simulink model "FF_statefbk"  (R2020b)
settings: Solver=ode45  StartTime=0.0  StopTime=10  RelTol=1e-3  EnableMultiTasking=on
values from neighbouring files (symbols this model uses):
  A = [0 1 ... (first row only)    [TestDIST_EFFECT_DCmotor_zp(1).m]    (also in TestDIST_EFFECT_DCmotor_zp.m; lqr_DOB_2_5.mat = [0  1; 0  0]; lqr_DOB_5.mat = [0  1; 0  0]; lqr_DOB_8.mat = [0  1; 0  0])
  B = [0; Kt/Rm/Jt]    [TestDIST_EFFECT_DCmotor_zp(1).m]    (also in TestDIST_EFFECT_DCmotor_zp.m; lqr_DOB_2_5.mat = [0 239.250934036]; lqr_DOB_5.mat = [0 239.250934036]; lqr_DOB_8.mat = [0 239.250934036])
  Jt = Jm+J1+J2    (= 2.089856e-05)    [TestDIST_EFFECT_DCmotor_zp(1).m]    (also in TestDIST_EFFECT_DCmotor_zp.m; lqr_DOB_2_5.mat; lqr_DOB_5.mat; lqr_DOB_8.mat)
  KK = dlqr(Fs,Gs,Q,R)    [TestDIST_EFFECT_DCmotor_zp(1).m]    (also in TestDIST_EFFECT_DCmotor_zp.m; lqr_DOB_2_5.mat = [27.9647466006 0.483496818901]; lqr_DOB_5.mat = [27.9647466006 0.483496818901]; lqr_DOB_8.mat = [27.9647466006 0.483496818901])
  Kt = 0.042    [TestDIST_EFFECT_DCmotor_zp(1).m]    (also in TestDIST_EFFECT_DCmotor_zp.m; lqr_DOB_2_5.mat; lqr_DOB_5.mat; lqr_DOB_8.mat)
  Rm = 8.4    [TestDIST_EFFECT_DCmotor_zp(1).m]    (also in TestDIST_EFFECT_DCmotor_zp.m; lqr_DOB_2_5.mat; lqr_DOB_5.mat; lqr_DOB_8.mat)
settings Model: Creator=oboe  LastModifiedBy=marco
settings DataIOCC: LimitDataPoints=on  SaveFormat=Array  ReturnWorkspaceOutputs=off
settings OptimizationCC: LifeSpan=inf
settings DebuggingCC: SolverPrmCheckMsg=warning  SFUnexpectedBacktrackingDiag=warning  SFNoUnconditionalDefaultTransitionDiag=warning  SFExecutionAtInitializationDiag=none  ArithmeticOperatorsInVariantConditions=warning
settings HardwareCC: ProdBitPerPointer=32  ProdBitPerSizeT=32  ProdBitPerPtrDiffT=32  ProdLargestAtomicFloat=None  ProdIntDivRoundTo=Undefined  ProdEndianess=Unspecified  ProdWordSize=32  ProdHWDeviceType=32-bit Generic
settings ModelReferenceCC: PropagateSignalLabelsOutOfModel=off
settings SFSimCC: SimUseLocalCustomCode=off  CustomCodeUndefinedFunction=UseInterfaceOnly
settings RTWCC: RTWUseLocalCustomCode=off
settings CodeAppCC: StateflowObjectComments=on
settings GRTTargetCC: TargetLangStandard=C89/C90 (ANSI)
settings ConfigComp: CovMetricSettings=dw  CovSaveCumulativeToWorkspaceVar=on  CovSaveSingleToWorkspaceVar=on  CovExternalEMLEnable=off  CovSFcnEnable=off

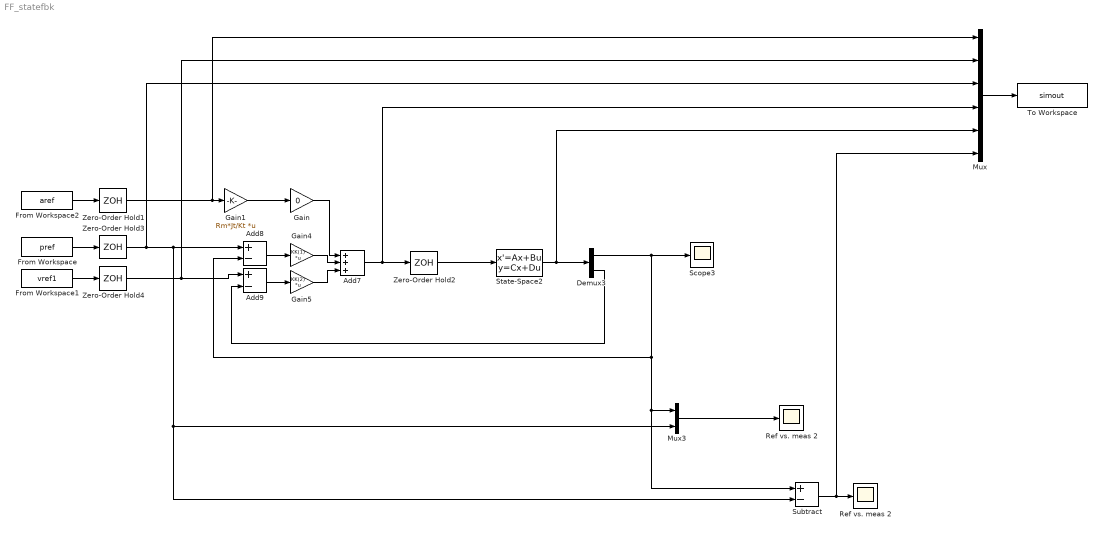
== system FF_statefbk ==
  Add7 : Sum  Inputs=+++
  Add8 : Sum  Inputs=+-
  Add9 : Sum  Inputs=+-
  Demux3 : Demux  Outputs=2
  From Workspace : FromWorkspace  VariableName=pref
  From Workspace1 : FromWorkspace  VariableName=vref1
  From Workspace2 : FromWorkspace  VariableName=aref
  Gain : Gain  Gain=0
  Gain1 : Gain  Gain=Rm*Jt/Kt  Multiplication=Matrix(K*u)
  Gain4 : Gain  Gain=KK(1)  Multiplication=Matrix(K*u)
  Gain5 : Gain  Gain=KK(2)  Multiplication=Matrix(K*u)
  Mux : Mux  Inputs=6
  Mux3 : Mux  Inputs=2
  Ref vs. meas 2 : Scope
  "Ref vs. meas 2 " : Scope
  Scope3 : Scope
  State-Space2 : StateSpace  A=A(1:2,1:2)  B=B(1:2)  C=eye(2)  D=[0;0]  InitialCondition=0
  Subtract : Sum  Inputs=+-
  To Workspace : ToWorkspace  VariableName=simout  SaveFormat=Structure With Time  SampleTime=-1
  Zero-Order Hold{1..4} (4 alike) : ZeroOrderHold  SampleTime=0.002
  wires:
  Mux3/1 -> "Ref vs. meas 2 "/1
  Zero-Order Hold2/1 -> State-Space2/1
  Demux3/1 -> Add8/2, Subtract/1, Mux3/1, Scope3/1
  Gain4/1 -> Add7/2
  Add7/1 -> Mux/4, Zero-Order Hold2/1
  Gain5/1 -> Add7/3
  State-Space2/1 -> Mux/5, Demux3/1
  Demux3/2 -> Add9/2
  Add9/1 -> Gain5/1
  Add8/1 -> Gain4/1
  From Workspace/1 -> Zero-Order Hold3/1
  Subtract/1 -> Mux/6, Ref vs. meas 2/1
  From Workspace1/1 -> Zero-Order Hold4/1
  From Workspace2/1 -> Zero-Order Hold1/1
  Gain1/1 -> Gain/1
  Gain/1 -> Add7/1
  Mux/1 -> To Workspace/1
  Zero-Order Hold1/1 -> Mux/1, Gain1/1
  Zero-Order Hold3/1 -> Mux/3, Add8/1, Mux3/2, Subtract/2
  Zero-Order Hold4/1 -> Mux/2, Add9/1
